simulink model "lab_one_task_one"  (R2018b)
settings: Solver=FixedStepDiscrete  StartTime=0.0  StopTime=10.0  RelTol=1e-3
settings Model: Creator=Romario  LastModifiedBy=Romario
settings OptimizationCC: DefaultParameterBehavior=Inlined  EnhancedBackFolding=on  PassReuseOutputArgsAs=Individual arguments  OptimizeBlockOrder=speed  DifferentSizesBufferReuse=on  OptimizationCustomize=off
settings DebuggingCC: UnderspecifiedInitializationDetection=Classic  MergeDetectMultiDrivingBlocksExec=none  ParameterTunabilityLossMsg=error
settings ModelReferenceCC: PropagateSignalLabelsOutOfModel=off
settings SFSimCC: MATLABDynamicMemAlloc=off
settings RTWCC: SystemTargetFile=ert.tlc  GenCodeOnly=on  TemplateMakefile=ert_default_tmf  GenerateReport=on  IncludeHyperlinkInReport=on  LaunchReport=on  GenerateTraceInfo=on  GenerateTraceReport=on  GenerateTraceReportSl=on  GenerateTraceReportSf=on  GenerateTraceReportEml=on
settings CodeAppCC: ForceParamTrailComments=on  IgnoreCustomStorageClasses=off  OperatorAnnotations=on  SimulinkDataObjDesc=on  SFDataObjDesc=on  InsertBlockDesc=on
settings ERTTargetCC: TargetLangStandard=C99 (ISO)  GenerateSampleERTMain=on  InlinedParameterPlacement=NonHierarchical  ERTCustomFileTemplate=example_file_process.tlc

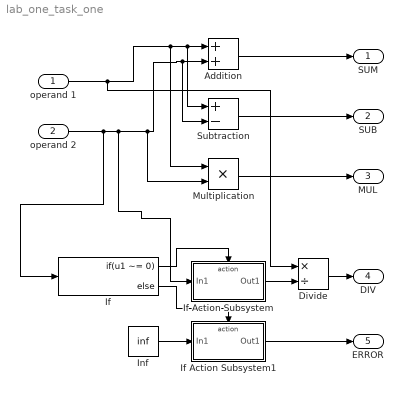
== system lab_one_task_one ==
  "operand 1 " : Inport
  operand 2 : Inport  Port=2
  Addition : Sum
  Divide : Product  Inputs=*/
  If : If  IfExpression=u1 ~= 0
  If Action Subsystem : Subsystem  TreatAsAtomicUnit=on
  If Action Subsystem1 : Subsystem  TreatAsAtomicUnit=on
  Inf : Constant  Value=inf  OutDataTypeStr=Inherit: Inherit via back propagation
  "Multiplication " : Product
  "Subtraction " : Sum  Inputs=+-
  SUM : Outport
  SUB : Outport  Port=2
  MUL : Outport  Port=3
  DIV : Outport  Port=4
  "ERROR " : Outport  Port=5  SignalName=ERROR
  wires:
  "operand 1 "/1 -> Divide/1, "Multiplication "/1, "Subtraction "/1, Addition/1
  Addition/1 -> SUM/1
  "Subtraction "/1 -> SUB/1
  "Multiplication "/1 -> MUL/1
  Divide/1 -> DIV/1
  If Action Subsystem/1(Out1) -> Divide/2
  If/1 -> If Action Subsystem/Action
  If/2 -> If Action Subsystem1/Action
  If Action Subsystem1/1(Out1) -> "ERROR "/1
  operand 2/1 -> If/1, If Action Subsystem/1(In1), "Multiplication "/2, "Subtraction "/2, Addition/2
  Inf/1 -> If Action Subsystem1/1(In1)

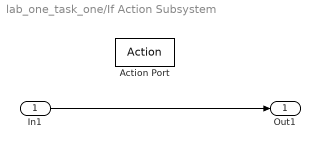
== system lab_one_task_one/If Action Subsystem ==
  In1 : Inport
  Action Port : ActionPort  ActionType=then
  Out1 : Outport
  wires:
  In1/1 -> Out1/1

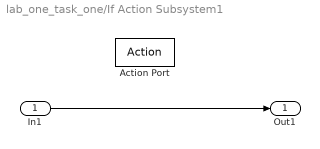
== system lab_one_task_one/If Action Subsystem1 ==
  In1 : Inport
  Action Port : ActionPort  ActionType=else
  Out1 : Outport
  wires:
  In1/1 -> Out1/1
